simulink model "MINI_BANSHEE_bckup"  (Simulink 8.1)
settings: Solver=ode1  StartTime=0.0  StopTime=inf  FixedStep=Ts  MaxStep=1e-3  RelTol=1e-3
PostLoadFcn:
  | BANSHEE_init;
InitFcn:
  | BANSHEE_init;
undefined symbols (not defined in the file): cable_spec, F1, F2, F3, fdesignblkfcn, gcbh, Left, SM_UtilityService, Ts, type, utility_service_lib, V
libraries: rtio_generic_modbus x37, relay_modbus_lib x36, cables_lib x17, breaker_lib x17, rtlab x15, rtio_opalrt_common x15, artemis x11, simulink x10, transformer_lib x7, simulink_extras x6, PQFV_lib x5, rtio_opalrt_op5142ex1 x4
(part 2 of 3)

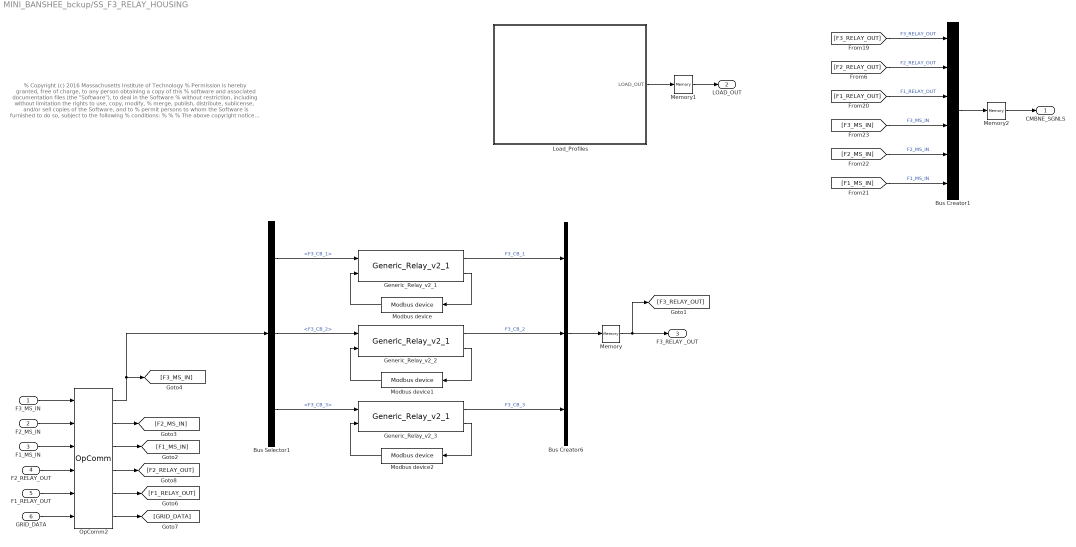
== system MINI_BANSHEE_bckup/SS_F3_RELAY_HOUSING ==
  note: % Copyright (c) 2016 Massachusetts Institute of Technology
      | % Permission is hereby granted, free of charge, to any person obtaining a copy of this
      | % software and associated documentation files (the "Software"), to deal in the Software
      | % without restriction, including without limitation the rights to use, copy, modify,
      | % merge, publish, distribute, sublicense, and/or sell copies of the Software, and to
      | % permit persons to whom the Software is furnished to do so, subject to the following
      | % conditions:
      | %
      | %
      | % The above copyright notice and this permission notice shall be included in
      | % all copies or substantial portions of the Software.
      | %
      | % THE SOFTWARE IS PROVIDED "AS IS", WITHOUT WARRANTY OF ANY KIND, EXPRESS OR IMPLIED,
      | % INCLUDING BUT NOT LIMITED TO THE WARRANTIES OF MERCHANTABILITY, FITNESS FOR A
      | % PARTICULAR PURPOSE AND NONINFRINGEMENT. IN NO EVENT SHALL THE AUTHORS OR COPYRIGHT
      | % HOLDERS BE LIABLE FOR ANY CLAIM, DAMAGES OR OTHER LIABILITY, WHETHER IN AN ACTION
      | % OF CONTRACT, TORT OR OTHERWISE, ARISING FROM, OUT OF OR IN CONNECTION WITH THE
      | % SOFTWARE OR THE USE OR OTHER DEALINGS IN THE SOFTWARE.
      | %
      | %
      | %%
  F3_MS_IN : Inport
  F2_MS_IN : Inport  Port=2
  F1_MS_IN : Inport  Port=3
  F2_RELAY_OUT : Inport  Port=4
  F1_RELAY_OUT : Inport  Port=5
  GRID_DATA : Inport  Port=6
  Bus Creator1 : BusCreator  Inputs=6
  Bus Creator6 : BusCreator  Inputs=3
  Bus Selector1 : BusSelector  OutputSignals=CB_DATA.F3_CB_1,CB_DATA.F3_CB_2,CB_DATA.F3_CB_3
  Generic_Relay_v2_1 : relay_modbus_lib/Generic_Relay_v2_1  Ts=Ts  relay_settings=[F3(1,:)]
  Generic_Relay_v2_2 : relay_modbus_lib/Generic_Relay_v2_1  Ts=Ts  relay_settings=[F3(2,:)]
  Generic_Relay_v2_3 : relay_modbus_lib/Generic_Relay_v2_1  Ts=Ts  relay_settings=[F3(3,:)]
  Load_Profiles : Subsystem
  Memory : Memory
  Memory1 : Memory
  Memory2 : Memory
  Modbus device : rtio_generic_modbus/Modbus device  conf_name=F3_relay_cfg1.opal  conf_name_mask=F3_relay_cfg1.xls  sample_time=Ts
  Modbus device1 : rtio_generic_modbus/Modbus device  conf_name=F3_relay_cfg2.opal  conf_name_mask=F3_relay_cfg2.xls  sample_time=Ts
  Modbus device2 : rtio_generic_modbus/Modbus device  conf_name=F3_relay_cfg3.opal  conf_name_mask=F3_relay_cfg3.xls  sample_time=Ts
  OpComm2 : rtlab/OpComm  nbport=6  groupe_acq=1  subsys_rate=0  st=0  Synchronization=on  Interpolation=on  Threshold=1.0  Missed_Data=off  Sim_Time=off  Samples=off  dynSigOut=off  from_console=0  warning_done=off  writeOpCommFile=off  Offset=off
  CMBNE_SGNLS : Outport
  LOAD_OUT : Outport  Port=2
  F3_RELAY _OUT : Outport  Port=3
  wires:
  Load_Profiles/1(LOAD_OUT) -> Memory1/1
  OpComm2/1 -> Bus Selector1/1, [F3_MS_IN]
  Generic_Relay_v2_1/2 -> Modbus device/1
  Modbus device/1 -> Generic_Relay_v2_1/2
  Generic_Relay_v2_2/2 -> Modbus device1/1
  Modbus device1/1 -> Generic_Relay_v2_2/2
  Modbus device2/1 -> Generic_Relay_v2_3/2
  Generic_Relay_v2_3/2 -> Modbus device2/1
  F3_MS_IN/1 -> OpComm2/1
  Bus Selector1/1 -> Generic_Relay_v2_1/1  "<F3_CB_1>"
  Bus Selector1/2 -> Generic_Relay_v2_2/1  "<F3_CB_2>"
  Bus Selector1/3 -> Generic_Relay_v2_3/1  "<F3_CB_3>"
  Generic_Relay_v2_1/1 -> Bus Creator6/1  "F3_CB_1"
  Generic_Relay_v2_2/1 -> Bus Creator6/2  "F3_CB_2"
  Generic_Relay_v2_3/1 -> Bus Creator6/3  "F3_CB_3"
  Bus Creator6/1 -> Memory/1
  Memory/1 -> [F3_RELAY_OUT], F3_RELAY _OUT/1
  Memory1/1 -> LOAD_OUT/1
  F2_RELAY_OUT/1 -> OpComm2/4
  F1_RELAY_OUT/1 -> OpComm2/5
  OpComm2/4 -> [F2_RELAY_OUT]
  OpComm2/5 -> [F1_RELAY_OUT]
  OpComm2/2 -> [F2_MS_IN]
  OpComm2/3 -> [F1_MS_IN]
  F2_MS_IN/1 -> OpComm2/2
  F1_MS_IN/1 -> OpComm2/3
  OpComm2/6 -> [GRID_DATA]
  GRID_DATA/1 -> OpComm2/6
  Memory2/1 -> CMBNE_SGNLS/1
  Bus Creator1/1 -> Memory2/1
  [F1_MS_IN] -> Bus Creator1/6  "F1_MS_IN"
  [F2_RELAY_OUT] -> Bus Creator1/2  "F2_RELAY_OUT"
  [F1_RELAY_OUT] -> Bus Creator1/3  "F1_RELAY_OUT"
  [F3_RELAY_OUT] -> Bus Creator1/1  "F3_RELAY_OUT"
  [F3_MS_IN] -> Bus Creator1/4  "F3_MS_IN"
  [F2_MS_IN] -> Bus Creator1/5  "F2_MS_IN"

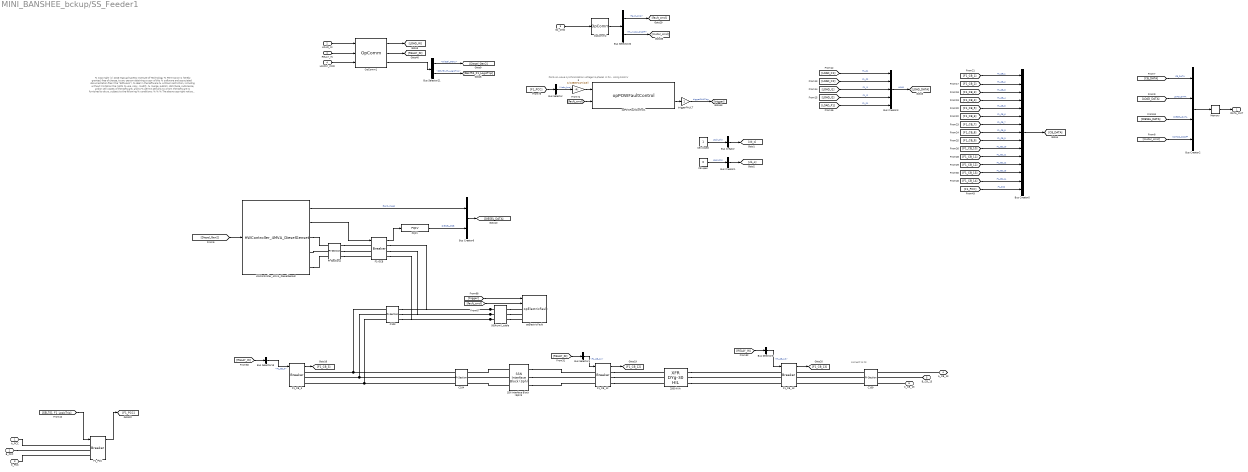
== system MINI_BANSHEE_bckup/SS_Feeder1 ==
  note: connect to F3
  note: % Copyright (c) 2016 Massachusetts Institute of Technology
      | % Permission is hereby granted, free of charge, to any person obtaining a copy of this
      | % software and associated documentation files (the "Software"), to deal in the Software
      | % without restriction, including without limitation the rights to use, copy, modify,
      | % merge, publish, distribute, sublicense, and/or sell copies of the Software, and to
      | % permit persons to whom the Software is furnished to do so, subject to the following
      | % conditions:
      | %
      | %
      | % The above copyright notice and this permission notice shall be included in
      | % all copies or substantial portions of the Software.
      | %
      | % THE SOFTWARE IS PROVIDED "AS IS", WITHOUT WARRANTY OF ANY KIND, EXPRESS OR IMPLIED,
      | % INCLUDING BUT NOT LIMITED TO THE WARRANTIES OF MERCHANTABILITY, FITNESS FOR A
      | % PARTICULAR PURPOSE AND NONINFRINGEMENT. IN NO EVENT SHALL THE AUTHORS OR COPYRIGHT
      | % HOLDERS BE LIABLE FOR ANY CLAIM, DAMAGES OR OTHER LIABILITY, WHETHER IN AN ACTION
      | % OF CONTRACT, TORT OR OTHERWISE, ARISING FROM, OUT OF OR IN CONNECTION WITH THE
      | % SOFTWARE OR THE USE OR OTHER DEALINGS IN THE SOFTWARE.
      | %
      | %
      | %%
  note: Point-on-wave synchronisation voltage (3-phase) in PU - Using 13.8 kV
  RELAY_IN : Inport
  LOAD_IN : Inport  Port=2
  SC_CMD : Inport  Port=3
  HWCtrl_CMD : Inport  Port=4
  2500 kVA : transformer_lib/XFR DYg-30 HIL  Rating=2500  Vp=13800  Vs=480  Z=5.75  XR=6.6
  500kcmil_cable : cables_lib/500kcmil_cable  length=1  par_sets=1
  Bus Creator : BusCreator  Inputs=1
  Bus Creator1 : BusCreator  Inputs=1
  Bus Creator2 : BusCreator
  Bus Creator3 : BusCreator  Inputs=5
  Bus Creator5 : BusCreator  Inputs=15
  Bus Creator6 : BusCreator  Inputs=2
  Bus Selector : BusSelector  OutputSignals=Vabc_bus
  Bus Selector1 : BusSelector  OutputSignals=F1_CB_12
  Bus Selector13 : BusSelector  OutputSignals=F1_CB_3
  Bus Selector20 : BusSelector  OutputSignals=fault_cmd,motor_ONOFF.F1_motor_ONOFF
  Bus Selector21 : BusSelector  OutputSignals=Diesel_Gen2,SEL751-F1_LogicTrip
  Bus Selector8 : BusSelector  OutputSignals=F1_CB_13
  C103 : cables_lib/PI-Section  cable_spec=[cable_spec(11, :)]  line_length=1000  parallel_sets=1
  C104 : cables_lib/PI-Section  cable_spec=[cable_spec(13, :)]  line_length=3000  parallel_sets=1
  C109 : cables_lib/PI-Section  cable_spec=[cable_spec(6, :)]  line_length=2000  parallel_sets=2
  CB closed : Constant
  CB open : Constant  Value=0
  F1-GCB : breaker_lib/Breaker  Ts=Ts  mech_delay=cb_mech_delay
  F1_CB_12 : breaker_lib/Breaker  Ts=Ts  mech_delay=cb_mech_delay
  F1_CB_13 : breaker_lib/Breaker  Ts=Ts  mech_delay=cb_mech_delay
  F1_CB_3 : breaker_lib/Breaker  Ts=Ts  mech_delay=cb_mech_delay
  F1_PCC : breaker_lib/Breaker  Ts=Ts  mech_delay=cb_mech_delay
  HWController_4MVA_DieselGenset : HWController_Diesel_GenSet_4MVA_lib/HWController_4MVA_DieselGenset
  Memory : Memory
  OpComm1 : rtlab/OpComm  nbport=3  groupe_acq=1  subsys_rate=0  st=0  Synchronization=on  Interpolation=on  Threshold=1.0  Missed_Data=off  Sim_Time=off  Samples=off  dynSigOut=off  from_console=0  warning_done=off  writeOpCommFile=off  Offset=off
  OpComm2 : rtlab/OpComm  nbport=1  groupe_acq=1  subsys_rate=0  st=0  Synchronization=on  Interpolation=on  Threshold=1.0  Missed_Data=off  Sim_Time=off  Samples=off  dynSigOut=off  from_console=1  warning_done=off  writeOpCommFile=off  Offset=off
  PI-Section4 : cables_lib/PI-Section  cable_spec=[cable_spec(11, :)]  line_length=2000  parallel_sets=1
  PQFV : PQFV_lib/PQFV  VRMSLL=13800
  SSN Interface Block (3ph)3 : ssn_lib/SSN Interface Block (3ph)  nb_phase=3  nb_port=2  p1_type=V-type(Left)  p2_type=V-type (Right)  p3_type=V-type(Left)  p4_type=V-type(Left)  p5_type=V-type(Left)  p6_type=V-type(Left)  p7_type=V-type(Left)  p8_type=V-type(Left)  p9_type=V-type(Left)  p10_type=V-type(Left)  p11_type=V-type(Left)  p12_type=V-type(Left)  p13_type=V-type(Left)  p14_type=V-type(Left)  p15_type=V-type(Left)  p16_type=V-type(Left)  I_port_shunt_resistance=1e9
  a : Gain  Gain=1/(13800*sqrt(2/3))
  opElectricFault : artemis/Tools /POW faults/opElectricFault  FaultLocation=location 2  FaultResistance=0.0001  GroundResistance=0.0001  InitialStates=[0 0 0]  SnubberResistance=1e6  SnubberCapacitance=inf
  opPOWFaultControl1 : artemis/Tools /POW faults/opPOWFaultControl  Ts=Ts  usePLL=off  Fgrid=60  PLL_k=[180 3200 1]  vol_sel=1: rising zero-corssing  SyncPhase_menu=A  T_acq=0.8
  triggerFAULT : Gain
  A_PCC : PMIOPort  Port=1  Side=Left
  B_PCC : PMIOPort  Port=2  Side=Left
  C_PCC : PMIOPort  Port=3  Side=Left
  A_CB_13 : PMIOPort  Port=4  Side=Right
  B_CB_13 : PMIOPort  Port=5  Side=Right
  C_CB_13 : PMIOPort  Port=6  Side=Right
  DATA_OUT : Outport
  wires:
  F1_PCC/1 -> [F1_PCC]
  Bus Creator/1 -> [cb_c]
  CB closed/1 -> Bus Creator/1  "Logic_trip"
  Bus Creator1/1 -> [cb_o]
  CB open/1 -> Bus Creator1/1  "Logic_trip"
  LOAD_IN/1 -> OpComm1/1
  OpComm1/1 -> [LOAD_IN]
  [LOAD_C1] -> Bus Creator3/1  "F1_C1"
  [LOAD_I2] -> Bus Creator3/4  "F1_I2"
  [LOAD_P1] -> Bus Creator3/5  "F1_P1"
  [LOAD_C2] -> Bus Creator3/2  "F1_C2"
  [LOAD_I1] -> Bus Creator3/3  "F1_I1"
  F1_CB_3/1 -> [F1_CB_3]
  F1_CB_12/1 -> [F1_CB_12]
  F1_CB_13/1 -> [F1_CB_13]
  [F1_CB_1] -> Bus Creator5/1  "F1_CB_1"
  [F1_CB_13] -> Bus Creator5/13  "F1_CB_13"
  [F1_CB_12] -> Bus Creator5/12  "F1_CB_12"
  [F1_CB_11] -> Bus Creator5/11  "F1_CB_11"
  [F1_CB_10] -> Bus Creator5/10  "F1_CB_10"
  [F1_CB_9] -> Bus Creator5/9  "F1_CB_9"
  [F1_CB_8] -> Bus Creator5/8  "F1_CB_8"
  [F1_CB_7] -> Bus Creator5/7  "F1_CB_7"
  [F1_CB_6] -> Bus Creator5/6  "F1_CB_6"
  [F1_CB_5] -> Bus Creator5/5  "F1_CB_5"
  [F1_CB_4] -> Bus Creator5/4  "F1_CB_4"
  [F1_CB_3] -> Bus Creator5/3  "F1_CB_3"
  [F1_CB_2] -> Bus Creator5/2  "F1_CB_2"
  RELAY_IN/1 -> OpComm1/2
  OpComm1/2 -> [RELAY_IN]
  Bus Selector13/1 -> F1_CB_3/1  "<F1_CB_3>"
  [RELAY_IN] -> Bus Selector13/1
  [RELAY_IN] -> Bus Selector1/1
  [RELAY_IN] -> Bus Selector8/1
  Bus Selector1/1 -> F1_CB_12/1  "<F1_CB_12>"
  Bus Selector8/1 -> F1_CB_13/1  "<F1_CB_13>"
  [F1_PCC] -> Bus Creator5/15  "F1_PCC"
  [F1_CB_14] -> Bus Creator5/14  "F1_CB_14"
  [fault_cmd] -> opPOWFaultControl1/2
  opPOWFaultControl1/2 -> triggerFAULT/1
  triggerFAULT/1 -> [trigger]  "triggerFAULTsig"
  [F1_PCC] -> Bus Selector/1
  Bus Selector/1 -> a/1  "<Vabc_bus>"
  a/1 -> opPOWFaultControl1/1
  SC_CMD/1 -> OpComm2/1
  [fault_cmd] -> opElectricFault/2
  [trigger] -> opElectricFault/1
  OpComm2/1 -> Bus Selector20/1
  Bus Selector20/1 -> [fault_cmd]  "<fault_cmd>"
  Bus Creator3/1 -> [LOAD_DATA]  "LOAD"
  Bus Creator5/1 -> [CB_DATA]
  [Diesel_Gen2] -> HWController_4MVA_DieselGenset/1
  HWController_4MVA_DieselGenset/2 -> F1-GCB/1
  OpComm1/3 -> Bus Selector21/1
  Bus Selector21/1 -> [Diesel_Gen2]  "<Diesel_Gen2>"
  HWCtrl_CMD/1 -> OpComm1/3
  F1-GCB/1 -> PQFV/1
  Bus Creator6/1 -> [DIESEL_DATA]
  PQFV/1 -> Bus Creator6/2  "DIESEL_GCB"
  HWController_4MVA_DieselGenset/1 -> Bus Creator6/1  "Gen2_meas"
  Memory/1 -> DATA_OUT/1
  Bus Creator2/1 -> Memory/1
  [CB_DATA] -> Bus Creator2/1  "CB_DATA"
  [LOAD_DATA] -> Bus Creator2/2  "LOAD_DATA"
  [DIESEL_DATA] -> Bus Creator2/3  "DIESEL_DATA"
  Bus Selector20/2 -> [motor_cmd]  "<F1_motor_ONOFF>"
  [motor_cmd] -> Bus Creator2/4  "MOTOR_ONOFF"
  Bus Selector21/2 -> [SEL751_F1_LogicTrip]  "<SEL751-F1_LogicTrip>"
  [SEL751_F1_LogicTrip] -> F1_PCC/1
  connections:
  2500 kVA/RConn2 -- F1_CB_13/LConn2
  F1_CB_12/RConn1 -- 2500 kVA/LConn1
  A_PCC/RConn1 -- F1_PCC/LConn1
  B_PCC/RConn1 -- F1_PCC/LConn2
  C104/LConn2 -- C103/LConn2 -- F1_CB_3/RConn2
  F1_CB_12/RConn2 -- 2500 kVA/LConn2
  F1_CB_12/RConn3 -- 2500 kVA/LConn3
  C104/LConn1 -- C103/LConn1 -- F1_CB_3/RConn1
  C104/LConn3 -- C103/LConn3 -- F1_CB_3/RConn3
  2500 kVA/RConn1 -- F1_CB_13/LConn1
  C_PCC/RConn1 -- F1_PCC/LConn3
  2500 kVA/RConn3 -- F1_CB_13/LConn3
  C109/LConn1 -- F1_CB_13/RConn1
  C109/LConn3 -- F1_CB_13/RConn3
  C109/LConn2 -- F1_CB_13/RConn2
  C_CB_13/RConn1 -- C109/RConn3
  B_CB_13/RConn1 -- C109/RConn2
  A_CB_13/RConn1 -- C109/RConn1
  SSN Interface Block (3ph)3/LConn2 -- C104/RConn2
  SSN Interface Block (3ph)3/LConn3 -- C104/RConn3
  SSN Interface Block (3ph)3/LConn1 -- C104/RConn1
  SSN Interface Block (3ph)3/RConn2 -- F1_CB_12/LConn2
  SSN Interface Block (3ph)3/RConn1 -- F1_CB_12/LConn1
  SSN Interface Block (3ph)3/RConn3 -- F1_CB_12/LConn3
  500kcmil_cable/RConn3 -- opElectricFault/LConn3
  500kcmil_cable/RConn1 -- opElectricFault/LConn1
  500kcmil_cable/RConn2 -- opElectricFault/LConn2
  500kcmil_cable/LConn3 -- C103/RConn3 -- F1-GCB/RConn3
  500kcmil_cable/LConn2 -- C103/RConn2 -- F1-GCB/RConn2
  500kcmil_cable/LConn1 -- C103/RConn1 -- F1-GCB/RConn1
  PI-Section4/RConn3 -- F1-GCB/LConn3
  PI-Section4/RConn1 -- F1-GCB/LConn1
  PI-Section4/RConn2 -- F1-GCB/LConn2
  HWController_4MVA_DieselGenset/RConn1 -- PI-Section4/LConn1
  HWController_4MVA_DieselGenset/RConn2 -- PI-Section4/LConn2
  HWController_4MVA_DieselGenset/RConn3 -- PI-Section4/LConn3

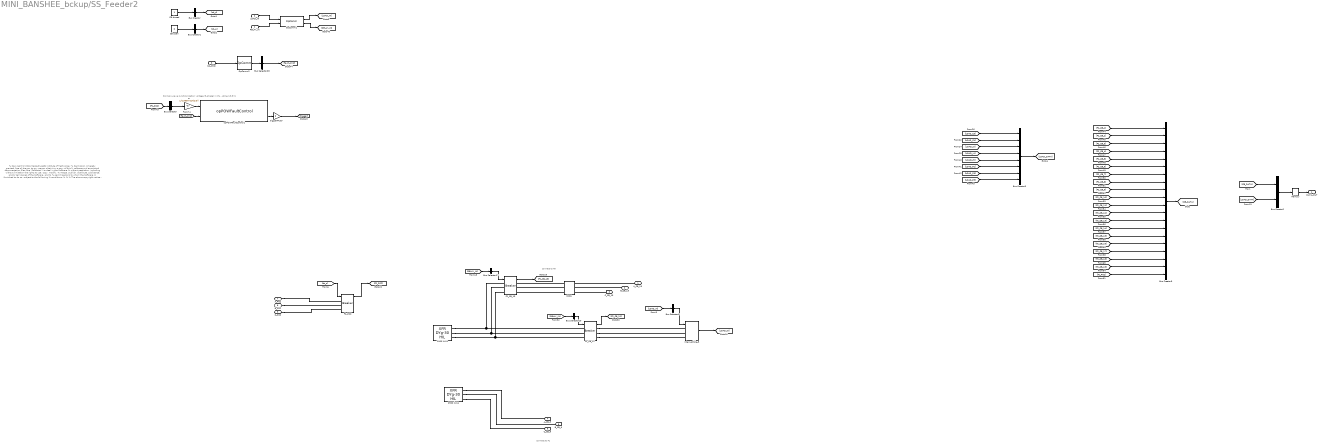
== system MINI_BANSHEE_bckup/SS_Feeder2 ==
  note: connect to F3
  note: connect to F1
  note: % Copyright (c) 2016 Massachusetts Institute of Technology
      | % Permission is hereby granted, free of charge, to any person obtaining a copy of this
      | % software and associated documentation files (the "Software"), to deal in the Software
      | % without restriction, including without limitation the rights to use, copy, modify,
      | % merge, publish, distribute, sublicense, and/or sell copies of the Software, and to
      | % permit persons to whom the Software is furnished to do so, subject to the following
      | % conditions:
      | %
      | %
      | % The above copyright notice and this permission notice shall be included in
      | % all copies or substantial portions of the Software.
      | %
      | % THE SOFTWARE IS PROVIDED "AS IS", WITHOUT WARRANTY OF ANY KIND, EXPRESS OR IMPLIED,
      | % INCLUDING BUT NOT LIMITED TO THE WARRANTIES OF MERCHANTABILITY, FITNESS FOR A
      | % PARTICULAR PURPOSE AND NONINFRINGEMENT. IN NO EVENT SHALL THE AUTHORS OR COPYRIGHT
      | % HOLDERS BE LIABLE FOR ANY CLAIM, DAMAGES OR OTHER LIABILITY, WHETHER IN AN ACTION
      | % OF CONTRACT, TORT OR OTHERWISE, ARISING FROM, OUT OF OR IN CONNECTION WITH THE
      | % SOFTWARE OR THE USE OR OTHER DEALINGS IN THE SOFTWARE.
      | %
      | %
      | %%
  note: Point-on-wave synchronisation voltage (3-phase) in PU - Using 13.8 kV
  RELAY_IN : Inport
  LOAD_IN : Inport  Port=2
  SC_CMD : Inport  Port=3
  1000 kVA1 : transformer_lib/XFR DYg-30 HIL  Rating=1000  Vp=13800  Vs=480  Z=5.56  XR=4.49
  2500 kVA1 : transformer_lib/XFR DYg-30 HIL  Rating=2500  Vp=13800  Vs=480  Z=5.56  XR=5.52
  Bus Creator : BusCreator  Inputs=1
  Bus Creator1 : BusCreator  Inputs=1
  Bus Creator2 : BusCreator  Inputs=2
  Bus Creator3 : BusCreator  Inputs=8
  Bus Creator5 : BusCreator  Inputs=20
  Bus Selector : BusSelector  OutputSignals=Vabc_bus
  Bus Selector17 : BusSelector  OutputSignals=F2_CB_13
  Bus Selector20 : BusSelector  OutputSignals=F2_CB_12
  Bus Selector28 : BusSelector  OutputSignals=fault_cmd
  Bus Selector5 : BusSelector  OutputSignals=I5
  C206 : cables_lib/PI-Section  cable_spec=[cable_spec(6, :)]  line_length=1500  parallel_sets=2
  CB closed : Constant
  CB open : Constant  Value=0
  F2_CB_12 : breaker_lib/Breaker  Ts=Ts  mech_delay=cb_mech_delay
  F2_CB_13 : breaker_lib/Breaker  Ts=Ts  mech_delay=cb_mech_delay
  F2_PCC : breaker_lib/Breaker  Ts=Ts  mech_delay=cb_mech_delay
  Interruptible_5 : Load_lib/Dynamic_Load  V=460  Ts=Ts
  Memory : Memory
  OpComm1 : rtlab/OpComm  nbport=2  groupe_acq=1  subsys_rate=0  st=0  Synchronization=on  Interpolation=on  Threshold=1.0  Missed_Data=off  Sim_Time=off  Samples=off  dynSigOut=off  from_console=0  warning_done=off  writeOpCommFile=off  Offset=off
  OpComm2 : rtlab/OpComm  nbport=1  groupe_acq=1  subsys_rate=0  st=0  Synchronization=on  Interpolation=on  Threshold=1.0  Missed_Data=off  Sim_Time=off  Samples=off  dynSigOut=off  from_console=1  warning_done=off  writeOpCommFile=off  Offset=off
  a : Gain  Gain=1/(13800*sqrt(2/3))
  opPOWFaultControl1 : artemis/Tools /POW faults/opPOWFaultControl  Ts=Ts  usePLL=off  Fgrid=60  PLL_k=[180 3200 1]  vol_sel=1: rising zero-corssing  SyncPhase_menu=A  T_acq=0.8
  triggerFAULT : Gain
  A_CB_13 : PMIOPort  Port=1  Side=Right
  B_CB_13 : PMIOPort  Port=2  Side=Right
  C_CB_13 : PMIOPort  Port=3  Side=Right
  A_CB_9 : PMIOPort  Port=4  Side=Right
  B_CB_9 : PMIOPort  Port=5  Side=Right
  C_CB_9 : PMIOPort  Port=6  Side=Right
  A_PCC : PMIOPort  Port=7  Side=Left
  B_PCC : PMIOPort  Port=8  Side=Left
  C_PCC : PMIOPort  Port=9  Side=Left
  DATA_OUT : Outport
  wires:
  [cb_c] -> F2_PCC/1
  Bus Creator/1 -> [cb_c]
  CB closed/1 -> Bus Creator/1  "Logic_trip"
  Bus Creator1/1 -> [cb_o]
  CB open/1 -> Bus Creator1/1  "Logic_trip"
  LOAD_IN/1 -> OpComm1/1
  OpComm1/1 -> [LOAD_IN]
  [LOAD_IN] -> Bus Selector5/1
  Bus Selector5/1 -> Interruptible_5/1  "<I5>"
  Interruptible_5/1 -> [LOAD_I5]
  [LOAD_C3] -> Bus Creator3/1  "F2_C3"
  Bus Creator3/1 -> [LOAD_DATA]  "LOAD"
  [LOAD_I4] -> Bus Creator3/4  "F2_I4"
  [LOAD_P2] -> Bus Creator3/6  "F2_P2"
  [LOAD_I5] -> Bus Creator3/5  "F2_I5"
  [LOAD_C4] -> Bus Creator3/2  "F2_C4"
  [LOAD_I3] -> Bus Creator3/3  "F2_I3"
  [LOAD_P3] -> Bus Creator3/7  "F2_P3"
  [LOAD_P5] -> Bus Creator3/8  "F2_P5"
  F2_CB_13/1 -> [F2_CB_13]
  [F2_CB_1] -> Bus Creator5/1  "F2_CB_1"
  [F2_CB_2] -> Bus Creator5/2  "F2_CB_2"
  [F2_CB_3] -> Bus Creator5/3  "F2_CB_3"
  [F2_CB_6] -> Bus Creator5/6  "F2_CB_6"
  [F2_CB_4] -> Bus Creator5/4  "F2_CB_4"
  [F2_CB_9] -> Bus Creator5/9  "F2_CB_9"
  [F2_CB_7] -> Bus Creator5/7  "F2_CB_7"
  [F2_CB_11] -> Bus Creator5/11  "F2_CB_11"
  [F2_CB_14] -> Bus Creator5/14  "F2_CB_14"
  [F2_CB_5] -> Bus Creator5/5  "F2_CB_5"
  [F2_CB_8] -> Bus Creator5/8  "F2_CB_8"
  [F2_CB_12] -> Bus Creator5/12  "F2_CB_12"
  [F2_CB_10] -> Bus Creator5/10  "F2_CB_10"
  [F2_CB_13] -> Bus Creator5/13  "F2_CB_13"
  [F2_CB_15] -> Bus Creator5/15  "F2_CB_15"
  [F2_CB_16] -> Bus Creator5/16  "F2_CB_16"
  RELAY_IN/1 -> OpComm1/2
  OpComm1/2 -> [RELAY_IN]
  [RELAY_IN] -> Bus Selector17/1
  [RELAY_IN] -> Bus Selector20/1
  Bus Selector17/1 -> F2_CB_13/1  "<F2_CB_13>"
  Bus Selector20/1 -> F2_CB_12/1  "<F2_CB_12>"
  [F2_CB_17] -> Bus Creator5/17  "F2_CB_17"
  F2_CB_12/1 -> [F2_CB_12]
  F2_PCC/1 -> [F2_PCC]
  [F2_PCC] -> Bus Creator5/20  "F2_PCC"
  [F2_CB_18] -> Bus Creator5/18  "F2_CB_18"
  [F2_CB_19] -> Bus Creator5/19  "F2_CB_19"
  [fault_cmd] -> opPOWFaultControl1/2
  opPOWFaultControl1/2 -> triggerFAULT/1
  triggerFAULT/1 -> [trigger]  "triggerFAULTsig"
  [F2_PCC] -> Bus Selector/1
  Bus Selector/1 -> a/1  "<Vabc_bus>"
  a/1 -> opPOWFaultControl1/1
  SC_CMD/1 -> OpComm2/1
  Memory/1 -> DATA_OUT/1
  OpComm2/1 -> Bus Selector28/1
  Bus Selector28/1 -> [fault_cmd]  "<fault_cmd>"
  Bus Creator2/1 -> Memory/1
  Bus Creator5/1 -> [CB_DATA]
  [CB_DATA] -> Bus Creator2/1  "CB_DATA"
  [LOAD_DATA] -> Bus Creator2/2  "LOAD_DATA"
  connections:
  F2_CB_13/LConn1 -- F2_CB_12/LConn1 -- 1000 kVA1/RConn1
  F2_CB_13/LConn2 -- 1000 kVA1/RConn2 -- F2_CB_12/LConn2
  F2_CB_13/LConn3 -- F2_CB_12/LConn3 -- 1000 kVA1/RConn3
  F2_CB_12/RConn3 -- Interruptible_5/LConn3
  F2_CB_12/RConn2 -- Interruptible_5/LConn2
  F2_CB_12/RConn1 -- Interruptible_5/LConn1
  C_PCC/RConn1 -- F2_PCC/LConn3
  B_PCC/RConn1 -- F2_PCC/LConn2
  A_PCC/RConn1 -- F2_PCC/LConn1
  2500 kVA1/RConn2 -- B_CB_9/RConn1
  2500 kVA1/RConn1 -- A_CB_9/RConn1
  2500 kVA1/RConn3 -- C_CB_9/RConn1
  C206/LConn3 -- F2_CB_13/RConn3
  C206/LConn2 -- F2_CB_13/RConn2
  C206/LConn1 -- F2_CB_13/RConn1
  C_CB_13/RConn1 -- C206/RConn3
  B_CB_13/RConn1 -- C206/RConn2
  A_CB_13/RConn1 -- C206/RConn1

== system MINI_BANSHEE_bckup/SC_ctrl/Overall ==
  F1 : Inport
  F2 : Inport  Port=2
  F3 : Inport  Port=3
  Iabc : Scope  NumInputPorts=3
      settings: ShowLegends=on  TimeRange=10  YMin=0~0~2  YMax=47.5~650~21  Decimation=10
  Vpu : Scope  NumInputPorts=3
      settings: ShowLegends=on  TimeRange=10  YMin=0.9975~1.0125~0.955  YMax=1.055~1.0675~1.06  SaveName=ScopeData3  Decimation=10
  currents : Subsystem
  voltages : Subsystem
  wires:
  voltages/1(oF1) -> Vpu/1
  voltages/2(oF2) -> Vpu/2
  voltages/3(oF3) -> Vpu/3
  currents/1(oF1) -> Iabc/1
  currents/2(oF2) -> Iabc/2
  currents/3(oF3) -> Iabc/3
  F3/1 -> voltages/3(F3), currents/3(F3)
  F2/1 -> currents/2(F2), voltages/2(F2)
  F1/1 -> voltages/1(F1), currents/1(F1)

== system MINI_BANSHEE_bckup/SC_ctrl/Status ==
  F1 : Inport
  F2 : Inport  Port=2
  F3 : Inport  Port=3
  Bus Selector : BusSelector  OutputSignals=F1_CB_1.m.status,F1_CB_2.m.status,F1_CB_3.m.status,F1_CB_4.m.status,F1_CB_5.m.status,F1_CB_6.m.status,F1_CB_7.m.status,F1_CB_8.m.status,F1_CB_9.m.status,F1_CB_10.m.status,F1_CB_11.m.status,F1_CB_12.m.status,F1_CB_13.m.status,F1_CB_14.m.status
  Bus Selector1 : BusSelector  OutputSignals=F2_CB_1.m.status,F2_CB_2.m.status,F2_CB_3.m.status,F2_CB_4.m.status,F2_CB_5.m.status,F2_CB_6.m.status,F2_CB_7.m.status,F2_CB_8.m.status,F2_CB_9.m.status,F2_CB_10.m.status,F2_CB_11.m.status,F2_CB_12.m.status,F2_CB_13.m.status,F2_CB_14.m.status,F2_CB_15.m.status,F2_CB_16.m.status,F2_CB_17.m.status,F2_CB_18.m.status,F2_CB_19.m.status
  Bus Selector2 : BusSelector  OutputSignals=F3_CB_1.m.status,F3_CB_2.m.status,F3_CB_3.m.status,F3_CB_4.m.status,F3_CB_5.m.status,F3_CB_6.m.status,F3_CB_7.m.status,F3_CB_8.m.status,F3_CB_9.m.status
  Mux : Mux  Inputs=14
  Mux1 : Mux  Inputs=19
  Mux2 : Mux  Inputs=9
  Status : Scope  NumInputPorts=3
      settings: ShowLegends=on  TimeRange=0.4  YMin=2~2~3  YMax=3~3~3  SaveName=ScopeData3  Decimation=20
  wires:
  Mux/1 -> Status/1  "F1"
  F1/1 -> Bus Selector/1
  Mux1/1 -> Status/2  "F2"
  F2/1 -> Bus Selector1/1
  Mux2/1 -> Status/3  "F3"
  F3/1 -> Bus Selector2/1
  Bus Selector1/3 -> Mux1/3  "<status>"
  Bus Selector1/13 -> Mux1/13  "<status>"
  Bus Selector1/8 -> Mux1/8  "<status>"
  Bus Selector1/4 -> Mux1/4  "<status>"
  Bus Selector1/6 -> Mux1/6  "<status>"
  Bus Selector1/2 -> Mux1/2  "<status>"
  Bus Selector1/7 -> Mux1/7  "<status>"
  Bus Selector1/10 -> Mux1/10  "<status>"
  Bus Selector1/12 -> Mux1/12  "<status>"
  Bus Selector1/1 -> Mux1/1  "<status>"
  Bus Selector1/5 -> Mux1/5  "<status>"
  Bus Selector1/14 -> Mux1/14  "<status>"
  Bus Selector1/9 -> Mux1/9  "<status>"
  Bus Selector1/11 -> Mux1/11  "<status>"
  Bus Selector1/17 -> Mux1/17  "<status>"
  Bus Selector1/16 -> Mux1/16  "<status>"
  Bus Selector1/15 -> Mux1/15  "<status>"
  Bus Selector1/18 -> Mux1/18  "<status>"
  Bus Selector1/19 -> Mux1/19  "<status>"
  Bus Selector/4 -> Mux/4  "<status>"
  Bus Selector/10 -> Mux/10  "<status>"
  Bus Selector/8 -> Mux/8  "<status>"
  Bus Selector/1 -> Mux/1  "<status>"
  Bus Selector/7 -> Mux/7  "<status>"
  Bus Selector/12 -> Mux/12  "<status>"
  Bus Selector/5 -> Mux/5  "<status>"
  Bus Selector/9 -> Mux/9  "<status>"
  Bus Selector/2 -> Mux/2  "<status>"
  Bus Selector/3 -> Mux/3  "<status>"
  Bus Selector/6 -> Mux/6  "<status>"
  Bus Selector/11 -> Mux/11  "<status>"
  Bus Selector/13 -> Mux/13  "<status>"
  Bus Selector/14 -> Mux/14  "<status>"
  Bus Selector2/6 -> Mux2/6  "<status>"
  Bus Selector2/5 -> Mux2/5  "<status>"
  Bus Selector2/7 -> Mux2/7  "<status>"
  Bus Selector2/4 -> Mux2/4  "<status>"
  Bus Selector2/8 -> Mux2/8  "<status>"
  Bus Selector2/3 -> Mux2/3  "<status>"
  Bus Selector2/9 -> Mux2/9  "<status>"
  Bus Selector2/2 -> Mux2/2  "<status>"
  Bus Selector2/1 -> Mux2/1  "<status>"

== system MINI_BANSHEE_bckup/SC_ctrl/Woodward ==
  16Din/16Dout GR3 : Subsystem
  Bus Creator2 : BusCreator  Inputs=1
  IOctrl : Outport
  wires:
  16Din/16Dout GR3/1(Dout) -> Bus Creator2/1  "16 DOUT GR3"
  Bus Creator2/1 -> IOctrl/1  "IO ctrl"

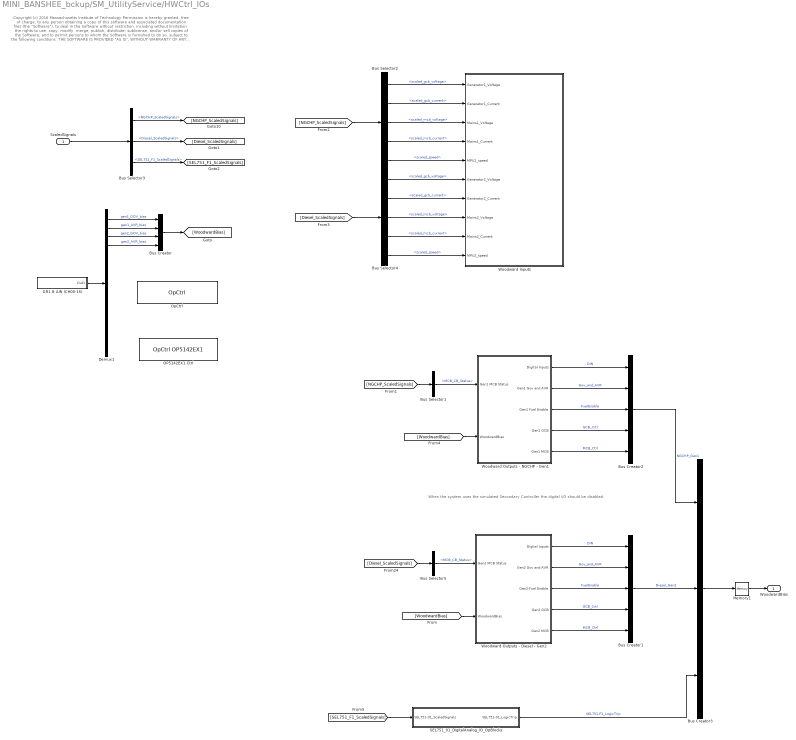
== system MINI_BANSHEE_bckup/SM_UtilityService/HWCtrl_IOs ==
  note: When the system uses the simulated
      | Secondary Controller the digital I/O
      | should be disabled.
  note: Copyright (c) 2016 Massachusetts Institute of Technology
      | Permission is hereby granted, free of charge, to any person obtaining a copy of this software and associated documentation files (the "Software"), to deal
      | in the Software without restriction, including without limitation the rights to use, copy, modify, merge, publish, distribute, sublicense, and/or sell copies of the
      | Software, and to permit persons to whom the Software is furnished to do so, subject to the following conditions:
      |
      | THE SOFTWARE IS PROVIDED "AS IS", WITHOUT WARRANTY OF ANY KIND, EXPRESS OR IMPLIED, INCLUDING BUT NOT LIMITED TO THE
      | WARRANTIES OF MERCHANTABILITY, FITNESS FOR A PARTICULAR PURPOSE AND NONINFRINGEMENT. IN NO EVENT SHALL THE AUTHORS
      | OR COPYRIGHT HOLDERS BE LIABLE FOR ANY CLAIM, DAMAGES OR OTHER LIABILITY, WHETHER IN AN ACTION OF CONTRACT, TORT OR
      | OTHERWISE, ARISING FROM, OUT OF OR IN CONNECTION WITH THE SOFTWARE OR THE USE OR OTHER DEALINGS IN THE SOFTWARE
  ScaledSignals : Inport
  Bus Creator : BusCreator
  Bus Creator1 : BusCreator  Inputs=5
  Bus Creator2 : BusCreator  Inputs=5
  Bus Creator3 : BusCreator  Inputs=3
  Bus Selector1 : BusSelector  OutputSignals=MCB_CB_Status
  Bus Selector2 : BusSelector  OutputSignals=scaled_gcb_voltage,scaled_gcb_current,scaled_mcb_voltage,scaled_mcb_current,scaled_speed
  Bus Selector3 : BusSelector  OutputSignals=NGCHP_ScaledSignals,Diesel_ScaledSignals,SEL751_F1_ScaledSignals
  Bus Selector4 : BusSelector  OutputSignals=scaled_gcb_voltage,scaled_gcb_current,scaled_mcb_voltage,scaled_mcb_current,scaled_speed
  Bus Selector5 : BusSelector  OutputSignals=MCB_CB_Status
  Demux1 : Demux  Outputs=16
  GR1 B AIN (CH00-15) : Subsystem
  Memory1 : Memory
  OP5142EX1 Ctrl : rtio_opalrt_op5142ex1/OpCtrl OP5142EX1  CtrlName='OP5142EX1 Ctrl'  boardid=1  BitstreamFilename=OP5142_1-EX-0000-2_3_4_54-16AIO_48AO_16DIO_16selDIO_CD-FF-01.bin  numconfig=-1  mode=Slave  externalClock=off  decimRtsi=0  calibIO=off  SampleTime=0  loadinport=-1
  OpCtrl : rtio_opalrt_common/OpCtrl  CtrlName='OpCtrl'  boardid=0  BitstreamFilename=VC707_2-EX-0001-2_3_2_20-48AIO16DIO16DIOSel-02-01.bin  numconfig=-1  mode=Master  externalClock=off  decimRtsi=0  calibIO=off  SampleTime=0  loadinport=-1  BoardType=VC707  SecondaryPresent=off  sync_type=Audio
  SEL751_01_DigitalAnalog_IO_OpBlocks : Subsystem
  Woodward Inputs : Subsystem
  Woodward Outputs - Diesel - Gen2 : Subsystem
  Woodward Outputs - NGCHP - Gen1 : Subsystem
  WoodwardBias : Outport
  wires:
  Bus Creator/1 -> [WoodwardBias]
  Memory1/1 -> WoodwardBias/1
  Bus Selector1/1 -> Woodward Outputs - NGCHP - Gen1/1(Gen1 MCB Status)  "<MCB_CB_Status>"
  [NGCHP_ScaledSignals] -> Bus Selector1/1
  [WoodwardBias] -> Woodward Outputs - NGCHP - Gen1/2(WoodwardBias)
  Woodward Outputs - NGCHP - Gen1/5(Gen1 MCB) -> Bus Creator2/5  "MCB_Ctrl"
  Woodward Outputs - Diesel - Gen2/1(Digital Inputs) -> Bus Creator1/1  "DIN"
  Woodward Outputs - NGCHP - Gen1/4(Gen1 GCB) -> Bus Creator2/4  "GCB_Crtl"
  Woodward Outputs - NGCHP - Gen1/3(Gen1 Fuel Enable) -> Bus Creator2/3  "FuelEnable"
  Woodward Outputs - NGCHP - Gen1/2(Gen1 Gov and AVR) -> Bus Creator2/2  "Gov_and_AVR"
  Woodward Outputs - NGCHP - Gen1/1(Digital Inputs) -> Bus Creator2/1  "DIN"
  Bus Creator2/1 -> Bus Creator3/1  "NGCHP_Gen1"
  Bus Creator3/1 -> Memory1/1
  Bus Creator1/1 -> Bus Creator3/2  "Diesel_Gen2"
  Woodward Outputs - Diesel - Gen2/5(Gen2 MCB) -> Bus Creator1/5  "MCB_Ctrl"
  Woodward Outputs - Diesel - Gen2/4(Gen2 GCB) -> Bus Creator1/4  "GCB_Crtl"
  Woodward Outputs - Diesel - Gen2/3(Gen2 Fuel Enable) -> Bus Creator1/3  "FuelEnable"
  Woodward Outputs - Diesel - Gen2/2(Gen2 Gov and AVR) -> Bus Creator1/2  "Gov_and_AVR"
  [Diesel_ScaledSignals] -> Bus Selector5/1
  [WoodwardBias] -> Woodward Outputs - Diesel - Gen2/2(WoodwardBias)
  Bus Selector5/1 -> Woodward Outputs - Diesel - Gen2/1(Gen2 MCB Status)  "<MCB_CB_Status>"
  Demux1/4 -> Bus Creator/4  "gen2_AVR_bias"
  Demux1/3 -> Bus Creator/3  "gen2_GOV_bias"
  Demux1/2 -> Bus Creator/2  "gen1_AVR_bias"
  Demux1/1 -> Bus Creator/1  "gen1_GOV_bias"
  GR1 B AIN (CH00-15)/1(Out1) -> Demux1/1
  Bus Selector4/5 -> Woodward Inputs/10(MPU2_speed)  "<scaled_speed>"
  Bus Selector4/4 -> Woodward Inputs/9(Mains2_Current)  "<scaled_mcb_current>"
  Bus Selector4/3 -> Woodward Inputs/8(Mains2_Voltage)  "<scaled_mcb_voltage>"
  Bus Selector4/2 -> Woodward Inputs/7(Generator2_Current)  "<scaled_gcb_current>"
  Bus Selector4/1 -> Woodward Inputs/6(Generator2_Voltage)  "<scaled_gcb_voltage>"
  [Diesel_ScaledSignals] -> Bus Selector4/1
  Bus Selector2/1 -> Woodward Inputs/1(Generator1_Voltage)  "<scaled_gcb_voltage>"
  Bus Selector2/2 -> Woodward Inputs/2(Generator1_Current)  "<scaled_gcb_current>"
  Bus Selector2/3 -> Woodward Inputs/3(Mains1_Voltage)  "<scaled_mcb_voltage>"
  Bus Selector2/4 -> Woodward Inputs/4(Mains1_Current)  "<scaled_mcb_current>"
  Bus Selector2/5 -> Woodward Inputs/5(MPU1_speed)  "<scaled_speed>"
  [NGCHP_ScaledSignals] -> Bus Selector2/1
  Bus Selector3/2 -> [Diesel_ScaledSignals]  "<Diesel_ScaledSignals>"
  Bus Selector3/1 -> [NGCHP_ScaledSignals]  "<NGCHP_ScaledSignals>"
  ScaledSignals/1 -> Bus Selector3/1
  SEL751_01_DigitalAnalog_IO_OpBlocks/1(SEL751-01_LogicTrip) -> Bus Creator3/3  "SEL751-F1_LogicTrip"
  [SEL751_F1_ScaledSignals] -> SEL751_01_DigitalAnalog_IO_OpBlocks/1(SEL751-01_ScaledSignals)
  Bus Selector3/3 -> [SEL751_F1_ScaledSignals]  "<SEL751_F1_ScaledSignals>"

== system MINI_BANSHEE_bckup/SS_F3/HWController_3.5MVA_NGCHP ==
  note: Copyright (c) 2016 Massachusetts Institute of Technology
      | Permission is hereby granted, free of charge, to any person obtaining a copy of this software and associated documentation files (the "Software"), to deal
      | in the Software without restriction, including without limitation the rights to use, copy, modify, merge, publish, distribute, sublicense, and/or sell copies of the
      | Software, and to permit persons to whom the Software is furnished to do so, subject to the following conditions:
      |
      | THE SOFTWARE IS PROVIDED "AS IS", WITHOUT WARRANTY OF ANY KIND, EXPRESS OR IMPLIED, INCLUDING BUT NOT LIMITED TO THE
      | WARRANTIES OF MERCHANTABILITY, FITNESS FOR A PARTICULAR PURPOSE AND NONINFRINGEMENT. IN NO EVENT SHALL THE AUTHORS
      | OR COPYRIGHT HOLDERS BE LIABLE FOR ANY CLAIM, DAMAGES OR OTHER LIABILITY, WHETHER IN AN ACTION OF CONTRACT, TORT OR
      | OTHERWISE, ARISING FROM, OUT OF OR IN CONNECTION WITH THE SOFTWARE OR THE USE OR OTHER DEALINGS IN THE SOFTWARE
  In1 : Inport
  In2 : Inport  Port=2
  HWControllerBias : Inport  Port=3
  Bus Creator2 : BusCreator  Inputs=6
  Bus Selector6 : BusSelector  OutputSignals=Heat Recovered; MBtu/hr
  Bus Selector7 : BusSelector  OutputSignals=TempActual,HeatFromBoiler MBtu/hr,CHPHeatContribution MBtu/hr,Thermal data.Heat Recovered; MBtu/hr,Thermal data.CO2 lbm/hr,Boiler_Nm^3/hr ,Boiler lbm/hr CO2
  CHPThermalModel : CHP_Model_lib/CHPThermalModel  SIM_HIL=SIM_HIL
  Demux : Demux  Outputs=2
  HWController_NG_Generator : HWController_NGCHP_Genset_3p5MVA_lib/HWController_NG_Generator
  Modbus device : rtio_generic_modbus/Modbus device  conf_name=CHP_slave_cfg.opal  conf_name_mask=CHP_slave_cfg.xls  sample_time=Ts
  Mux1 : Mux  Inputs=7
  A : PMIOPort  Tag=A  Port=1  Side=Right
      settings: AttributesFormatString=A
  B : PMIOPort  Port=2  Side=Right
  C : PMIOPort  Port=3  Side=Right
  Out1 : Outport
  Generator Data : Outport  Port=2
  GCB Control : Outport  Port=3
  wires:
  Bus Selector7/6 -> Mux1/6  "<Boiler_Nm^3/hr >"
  Bus Selector7/7 -> Mux1/7  "<Boiler lbm/hr CO2 >"
  CHPThermalModel/5 -> Bus Creator2/6
  CHPThermalModel/4 -> Bus Creator2/5
  HWControllerBias/1 -> HWController_NG_Generator/1
  HWController_NG_Generator/3 -> [HeatRec_MBtuhr]  "Thermal data"
  Bus Selector7/3 -> Mux1/3  "<CHPHeatContribution MBtu/hr>"
  CHPThermalModel/1 -> Bus Creator2/2  "TempActual"
  Demux/2 -> CHPThermalModel/4
  CHPThermalModel/2 -> Bus Creator2/3
  Bus Selector7/2 -> Mux1/2  "<HeatFromBoiler MBtu/hr>"
  Bus Selector7/5 -> Mux1/5  "<CO2 lbm/hr>"
  Bus Selector7/4 -> Mux1/4  "<Heat Recovered; MBtu/hr>"
  Bus Selector7/1 -> Mux1/1  "<TempActual>"
  In1/1 -> CHPThermalModel/2
  Mux1/1 -> Modbus device/4
  Demux/1 -> CHPThermalModel/3
  CHPThermalModel/3 -> Bus Creator2/4
  [HeatRec_MBtuhr] -> Bus Selector6/1, Bus Creator2/1  "Thermal data"
  Modbus device/2 -> Demux/1
  HWController_NG_Generator/1 -> Generator Data/1
  HWController_NG_Generator/2 -> GCB Control/1
  Bus Selector6/1 -> CHPThermalModel/1  "<Heat Recovered; MBtu/hr>"
  Bus Creator2/1 -> Out1/1, Bus Selector7/1  "CHPData"
  In2/1 -> CHPThermalModel/5  "CHP_SIM_Cmds"
  connections:
  HWController_NG_Generator/RConn3 -- C/RConn1
  HWController_NG_Generator/RConn2 -- B/RConn1
  HWController_NG_Generator/RConn1 -- A/RConn1

== system MINI_BANSHEE_bckup/SS_F3_RELAY_HOUSING/Load_Profiles ==
  note: % Copyright (c) 2016 Massachusetts Institute of Technology
      | % Permission is hereby granted, free of charge, to any person obtaining a copy of this
      | % software and associated documentation files (the "Software"), to deal in the Software
      | % without restriction, including without limitation the rights to use, copy, modify,
      | % merge, publish, distribute, sublicense, and/or sell copies of the Software, and to
      | % permit persons to whom the Software is furnished to do so, subject to the following
      | % conditions:
      | %
      | %
      | % The above copyright notice and this permission notice shall be included in
      | % all copies or substantial portions of the Software.
      | %
      | % THE SOFTWARE IS PROVIDED "AS IS", WITHOUT WARRANTY OF ANY KIND, EXPRESS OR IMPLIED,
      | % INCLUDING BUT NOT LIMITED TO THE WARRANTIES OF MERCHANTABILITY, FITNESS FOR A
      | % PARTICULAR PURPOSE AND NONINFRINGEMENT. IN NO EVENT SHALL THE AUTHORS OR COPYRIGHT
      | % HOLDERS BE LIABLE FOR ANY CLAIM, DAMAGES OR OTHER LIABILITY, WHETHER IN AN ACTION
      | % OF CONTRACT, TORT OR OTHERWISE, ARISING FROM, OUT OF OR IN CONNECTION WITH THE
      | % SOFTWARE OR THE USE OR OTHER DEALINGS IN THE SOFTWARE.
      | %
      | %
      | %%
  note: Stop_index = length of data - 1 to data chopping
  Bus Creator2 : BusCreator  Inputs=2
  Demux1 : Demux  Outputs=6
  Demux2 : Demux  Outputs=6
  "Interpolation " : Constant
  Mux : Mux  Inputs=6
  OpFromFile : rtlab/DataLogging/OpFromFile  filename_mode=Static (same filename all the time)  reload_mode=Next time model is paused (Real-Time)  init_file_id=0  filename=NONSHEDDABLE.mat  rtpath='./'  nrtpath='.\'  sample_time=0
  OpFromFile1 : rtlab/DataLogging/OpFromFile  filename_mode=Static (same filename all the time)  reload_mode=Next time model is paused (Real-Time)  init_file_id=0  filename=SHEDDABLE.mat  rtpath='./'  nrtpath='.\'  sample_time=0
  "Repetative " : Constant
  "Start_Index " : Constant
  "State " : Constant
  "Stop_Index " : Constant  Value=2000-1
  "Time_Scale_Factor " : Constant
  LOAD_OUT : Outport
  wires:
  Mux/1 -> Demux2/1, Demux1/1
  Bus Creator2/1 -> LOAD_OUT/1
  Demux1/1 -> OpFromFile/1
  Demux1/2 -> OpFromFile/2
  Demux1/3 -> OpFromFile/3
  Demux2/6 -> OpFromFile1/6
  Demux2/4 -> OpFromFile1/4
  Demux2/3 -> OpFromFile1/3
  Demux1/4 -> OpFromFile/4
  Demux2/5 -> OpFromFile1/5
  Demux2/2 -> OpFromFile1/2
  Demux2/1 -> OpFromFile1/1
  Demux1/5 -> OpFromFile/5
  Demux1/6 -> OpFromFile/6
  "Repetative "/1 -> Mux/2
  "State "/1 -> Mux/1
  OpFromFile/2 -> Bus Creator2/1  "NONSHEDDABLE"
  "Start_Index "/1 -> Mux/3
  OpFromFile1/2 -> Bus Creator2/2  "SHEDDABLE"
  "Time_Scale_Factor "/1 -> Mux/5
  "Stop_Index "/1 -> Mux/4
  "Interpolation "/1 -> Mux/6

== system MINI_BANSHEE_bckup/SC_ctrl/Overall/currents ==
  F1 : Inport
  F2 : Inport  Port=2
  F3 : Inport  Port=3
  1ph_rms1 : Subsystem
  1ph_rms10 : Subsystem
  1ph_rms11 : Subsystem
  1ph_rms12 : Subsystem
  1ph_rms13 : Subsystem
  1ph_rms14 : Subsystem
  1ph_rms15 : Subsystem
  1ph_rms2 : Subsystem
  1ph_rms3 : Subsystem
  1ph_rms4 : Subsystem
  1ph_rms5 : Subsystem
  1ph_rms6 : Subsystem
  1ph_rms7 : Subsystem
  1ph_rms8 : Subsystem
  1ph_rms9 : Subsystem
  Bus Selector : BusSelector  OutputSignals=F1_CB_1.m.Iabc,F1_CB_2.m.Iabc,F1_CB_3.m.Iabc,F1_CB_6.m.Iabc,F1_CB_10.m.Iabc
  Bus Selector1 : BusSelector  OutputSignals=F2_CB_1.m.Iabc,F2_CB_2.m.Iabc,F2_CB_3.m.Iabc,F2_CB_7.m.Iabc,F2_CB_14.m.Iabc,F2_CB_15.m.Iabc
  Bus Selector2 : BusSelector  OutputSignals=F3_CB_1.m.Iabc,F3_CB_2.m.Iabc,F3_CB_3.m.Iabc,F3_CB_4.m.Iabc
  Mux : Mux  Inputs=5
  Mux1 : Mux  Inputs=6
  Mux2 : Mux
  RMS_Calculator : Subsystem
  RMS_Calculator1 : Subsystem
  RMS_Calculator2 : Subsystem
  oF1 : Outport
  oF2 : Outport  Port=2
  oF3 : Outport  Port=3
  wires:
  Mux/1 -> RMS_Calculator/1(Signal)  "F1"
  Mux1/1 -> RMS_Calculator1/1(Signal)  "F2"
  Mux2/1 -> RMS_Calculator2/1(Signal)  "F3"
  Bus Selector/5 -> 1ph_rms3/1(i)  "<Iabc>"
  Bus Selector/4 -> 1ph_rms4/1(i)  "<Iabc>"
  Bus Selector/3 -> 1ph_rms2/1(i)  "<Iabc>"
  Bus Selector/2 -> 1ph_rms1/1(i)  "<Iabc>"
  Bus Selector/1 -> 1ph_rms6/1(i)  "<Iabc>"
  Bus Selector1/4 -> 1ph_rms9/1(i)  "<Iabc>"
  Bus Selector1/5 -> 1ph_rms13/1(i)  "<Iabc>"
  Bus Selector1/3 -> 1ph_rms8/1(i)  "<Iabc>"
  Bus Selector1/6 -> 1ph_rms10/1(i)  "<Iabc>"
  Bus Selector1/2 -> 1ph_rms7/1(i)  "<Iabc>"
  Bus Selector1/1 -> 1ph_rms5/1(i)  "<Iabc>"
  Bus Selector2/4 -> 1ph_rms15/1(i)  "<Iabc>"
  Bus Selector2/2 -> 1ph_rms12/1(i)  "<Iabc>"
  Bus Selector2/3 -> 1ph_rms11/1(i)  "<Iabc>"
  Bus Selector2/1 -> 1ph_rms14/1(i)  "<Iabc>"
  1ph_rms6/1(o) -> Mux/1
  1ph_rms1/1(o) -> Mux/2
  1ph_rms2/1(o) -> Mux/3
  1ph_rms3/1(o) -> Mux/5
  1ph_rms4/1(o) -> Mux/4
  1ph_rms5/1(o) -> Mux1/1
  1ph_rms7/1(o) -> Mux1/2
  1ph_rms8/1(o) -> Mux1/3
  1ph_rms9/1(o) -> Mux1/4
  1ph_rms14/1(o) -> Mux2/1
  1ph_rms13/1(o) -> Mux1/5
  1ph_rms10/1(o) -> Mux1/6
  1ph_rms12/1(o) -> Mux2/2
  1ph_rms11/1(o) -> Mux2/3
  1ph_rms15/1(o) -> Mux2/4
  RMS_Calculator/1(RMS_Signal) -> oF1/1
  RMS_Calculator1/1(RMS_Signal) -> oF2/1
  RMS_Calculator2/1(RMS_Signal) -> oF3/1
  F1/1 -> Bus Selector/1
  F2/1 -> Bus Selector1/1
  F3/1 -> Bus Selector2/1

== system MINI_BANSHEE_bckup/SC_ctrl/Overall/voltages ==
  F1 : Inport
  F2 : Inport  Port=2
  F3 : Inport  Port=3
  Bus Selector : BusSelector  OutputSignals=F1_CB_1.m.Vpu,F1_CB_2.m.Vpu,F1_CB_3.m.Vpu,F1_CB_4.m.Vpu,F1_CB_5.m.Vpu,F1_CB_6.m.Vpu,F1_CB_7.m.Vpu,F1_CB_8.m.Vpu,F1_CB_9.m.Vpu,F1_CB_10.m.Vpu,F1_CB_11.m.Vpu,F1_CB_12.m.Vpu,F1_CB_13.m.Vpu,F1_CB_14.m.Vpu
  Bus Selector1 : BusSelector  OutputSignals=F2_CB_1.m.Vpu,F2_CB_2.m.Vpu,F2_CB_3.m.Vpu,F2_CB_4.m.Vpu,F2_CB_5.m.Vpu,F2_CB_6.m.Vpu,F2_CB_7.m.Vpu,F2_CB_8.m.Vpu,F2_CB_9.m.Vpu,F2_CB_10.m.Vpu,F2_CB_11.m.Vpu,F2_CB_12.m.Vpu,F2_CB_13.m.Vpu,F2_CB_14.m.Vpu,F2_CB_15.m.Vpu,F2_CB_16.m.Vpu,F2_CB_17.m.Vpu,F2_CB_18.m.Vpu,F2_CB_19.m.Vpu
  Bus Selector2 : BusSelector  OutputSignals=F3_CB_1.m.Vpu,F3_CB_2.m.Vpu,F3_CB_3.m.Vpu,F3_CB_4.m.Vpu,F3_CB_5.m.Vpu,F3_CB_6.m.Vpu,F3_CB_7.m.Vpu,F3_CB_8.m.Vpu,F3_CB_9.m.Vpu
  Mux : Mux  Inputs=14
  Mux1 : Mux  Inputs=19
  Mux2 : Mux  Inputs=9
  oF1 : Outport
  oF2 : Outport  Port=2
  oF3 : Outport  Port=3
  wires:
  Mux/1 -> oF1/1  "F1"
  F1/1 -> Bus Selector/1
  Mux1/1 -> oF2/1  "F2"
  F2/1 -> Bus Selector1/1
  Mux2/1 -> oF3/1  "F3"
  F3/1 -> Bus Selector2/1
  Bus Selector/14 -> Mux/14  "<Vpu>"
  Bus Selector/6 -> Mux/6  "<Vpu>"
  Bus Selector/5 -> Mux/5  "<Vpu>"
  Bus Selector/10 -> Mux/10  "<Vpu>"
  Bus Selector/4 -> Mux/4  "<Vpu>"
  Bus Selector/9 -> Mux/9  "<Vpu>"
  Bus Selector/7 -> Mux/7  "<Vpu>"
  Bus Selector/2 -> Mux/2  "<Vpu>"
  Bus Selector/1 -> Mux/1  "<Vpu>"
  Bus Selector/3 -> Mux/3  "<Vpu>"
  Bus Selector/13 -> Mux/13  "<Vpu>"
  Bus Selector/12 -> Mux/12  "<Vpu>"
  Bus Selector/11 -> Mux/11  "<Vpu>"
  Bus Selector/8 -> Mux/8  "<Vpu>"
  Bus Selector1/19 -> Mux1/19  "<Vpu>"
  Bus Selector1/18 -> Mux1/18  "<Vpu>"
  Bus Selector1/7 -> Mux1/7  "<Vpu>"
  Bus Selector1/10 -> Mux1/10  "<Vpu>"
  Bus Selector1/11 -> Mux1/11  "<Vpu>"
  Bus Selector1/2 -> Mux1/2  "<Vpu>"
  Bus Selector1/13 -> Mux1/13  "<Vpu>"
  Bus Selector1/14 -> Mux1/14  "<Vpu>"
  Bus Selector1/15 -> Mux1/15  "<Vpu>"
  Bus Selector1/6 -> Mux1/6  "<Vpu>"
  Bus Selector1/4 -> Mux1/4  "<Vpu>"
  Bus Selector1/3 -> Mux1/3  "<Vpu>"
  Bus Selector1/1 -> Mux1/1  "<Vpu>"
  Bus Selector1/5 -> Mux1/5  "<Vpu>"
  Bus Selector1/8 -> Mux1/8  "<Vpu>"
  Bus Selector1/12 -> Mux1/12  "<Vpu>"
  Bus Selector1/16 -> Mux1/16  "<Vpu>"
  Bus Selector1/17 -> Mux1/17  "<Vpu>"
  Bus Selector1/9 -> Mux1/9  "<Vpu>"
  Bus Selector2/5 -> Mux2/5  "<Vpu>"
  Bus Selector2/4 -> Mux2/4  "<Vpu>"
  Bus Selector2/6 -> Mux2/6  "<Vpu>"
  Bus Selector2/3 -> Mux2/3  "<Vpu>"
  Bus Selector2/7 -> Mux2/7  "<Vpu>"
  Bus Selector2/8 -> Mux2/8  "<Vpu>"
  Bus Selector2/2 -> Mux2/2  "<Vpu>"
  Bus Selector2/9 -> Mux2/9  "<Vpu>"
  Bus Selector2/1 -> Mux2/1  "<Vpu>"

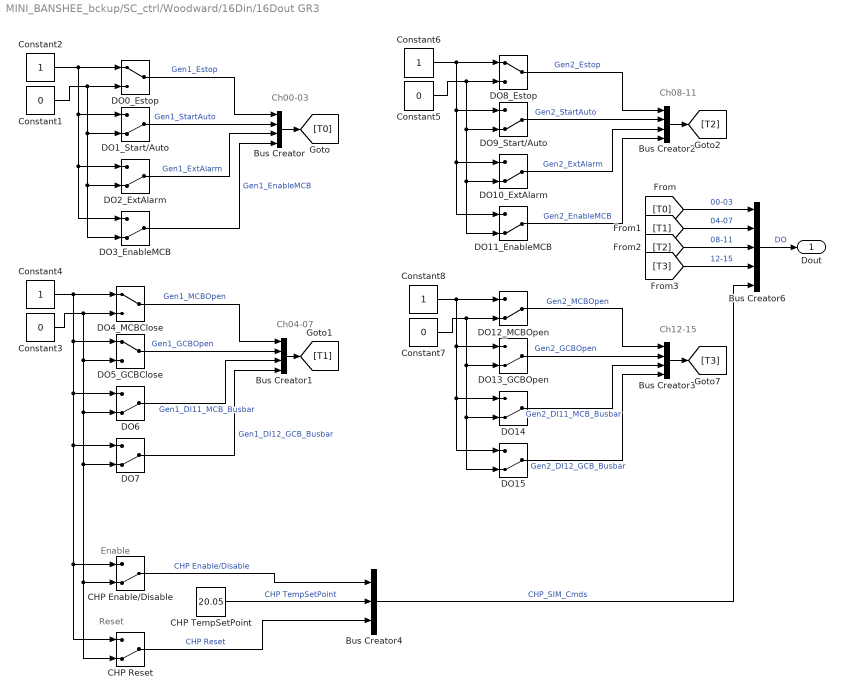
== system MINI_BANSHEE_bckup/SC_ctrl/Woodward/16Din/16Dout GR3 ==
  note: Ch00-03
  note: Ch04-07
  note: Ch08-11
  note: Ch12-15
  note: Enable
  note: Reset
  Bus Creator{,1..3} (4 alike) : BusCreator
  Bus Creator4 : BusCreator  Inputs=3
  Bus Creator6 : BusCreator  Inputs=5
  CHP Enable/Disable : ManualSwitch  CurrentSetting=0
  CHP Reset : ManualSwitch  CurrentSetting=0
  CHP TempSetPoint : Constant  Value=20.05
  Constant{1,3,5,7} (4 alike) : Constant  Value=0
  Constant{2,4,6,8} (4 alike) : Constant
  DO0_Estop : ManualSwitch
  DO10_ExtAlarm : ManualSwitch  CurrentSetting=0
  DO11_EnableMCB : ManualSwitch  CurrentSetting=0
  DO12_MCBOpen : ManualSwitch  CurrentSetting=0
  DO13_GCBOpen : ManualSwitch  CurrentSetting=0
  DO{6..7,14..15} (4 alike) : ManualSwitch  CurrentSetting=0
  DO1_Start/Auto : ManualSwitch  CurrentSetting=0
  DO2_ExtAlarm : ManualSwitch  CurrentSetting=0
  DO3_EnableMCB : ManualSwitch  CurrentSetting=0
  DO4_MCBClose : ManualSwitch
  DO5_GCBClose : ManualSwitch
  DO8_Estop : ManualSwitch
  DO9_Start/Auto : ManualSwitch  CurrentSetting=0
  Dout : Outport
  wires:
  Bus Creator4/1 -> Bus Creator6/5  "CHP_SIM_Cmds"
  CHP Reset/1 -> Bus Creator4/3  "CHP Reset"
  CHP TempSetPoint/1 -> Bus Creator4/2  "CHP TempSetPoint"
  CHP Enable/Disable/1 -> Bus Creator4/1  "CHP Enable/Disable"
  Bus Creator6/1 -> Dout/1  "DO"
  Constant2/1 -> DO0_Estop/1, DO1_Start/Auto/1, DO3_EnableMCB/1, DO2_ExtAlarm/1
  Constant1/1 -> DO0_Estop/2, DO1_Start/Auto/2, DO3_EnableMCB/2, DO2_ExtAlarm/2
  DO0_Estop/1 -> Bus Creator/1  "Gen1_Estop"
  DO1_Start/Auto/1 -> Bus Creator/2  "Gen1_StartAuto"
  DO2_ExtAlarm/1 -> Bus Creator/3  "Gen1_ExtAlarm"
  DO3_EnableMCB/1 -> Bus Creator/4  "Gen1_EnableMCB"
  Constant4/1 -> DO6/1, DO7/1, CHP Enable/Disable/1, CHP Reset/1, DO5_GCBClose/1, DO4_MCBClose/1
  Constant3/1 -> DO6/2, CHP Enable/Disable/2, CHP Reset/2, DO7/2, DO5_GCBClose/2, DO4_MCBClose/2
  DO4_MCBClose/1 -> Bus Creator1/1  "Gen1_MCBOpen"
  DO5_GCBClose/1 -> Bus Creator1/2  "Gen1_GCBOpen"
  DO6/1 -> Bus Creator1/3  "Gen1_DI11_MCB_Busbar"
  DO7/1 -> Bus Creator1/4  "Gen1_DI12_GCB_Busbar"
  Constant6/1 -> DO8_Estop/1, DO9_Start/Auto/1, DO11_EnableMCB/1, DO10_ExtAlarm/1
  Constant5/1 -> DO8_Estop/2, DO9_Start/Auto/2, DO11_EnableMCB/2, DO10_ExtAlarm/2
  DO8_Estop/1 -> Bus Creator2/1  "Gen2_Estop"
  DO9_Start/Auto/1 -> Bus Creator2/2  "Gen2_StartAuto"
  DO10_ExtAlarm/1 -> Bus Creator2/3  "Gen2_ExtAlarm"
  DO11_EnableMCB/1 -> Bus Creator2/4  "Gen2_EnableMCB"
  Constant8/1 -> DO14/1, DO15/1, DO13_GCBOpen/1, DO12_MCBOpen/1
  Constant7/1 -> DO14/2, DO15/2, DO13_GCBOpen/2, DO12_MCBOpen/2
  DO12_MCBOpen/1 -> Bus Creator3/1  "Gen2_MCBOpen"
  DO13_GCBOpen/1 -> Bus Creator3/2  "Gen2_GCBOpen"
  DO14/1 -> Bus Creator3/3  "Gen2_DI11_MCB_Busbar"
  DO15/1 -> Bus Creator3/4  "Gen2_DI12_GCB_Busbar"
  Bus Creator/1 -> [T0]
  Bus Creator1/1 -> [T1]
  Bus Creator3/1 -> [T3]
  Bus Creator2/1 -> [T2]
  [T0] -> Bus Creator6/1  "00-03"
  [T1] -> Bus Creator6/2  "04-07"
  [T2] -> Bus Creator6/3  "08-11"
  [T3] -> Bus Creator6/4  "12-15"

== system MINI_BANSHEE_bckup/SM_UtilityService/HWCtrl_IOs/GR1 B AIN (CH00-15) ==
  AnalogIn : rtio_opalrt_common/AnalogIn  CtrlName='OpCtrl'  portNb=1  FcnNos=Slot 1 Module B Subsection 1  size=16  maxcount=8  count=8  numchan=8  sampleTime=0
      settings: AttributesFormatString=%<CtrlName>
  AnalogIn1 : rtio_opalrt_common/AnalogIn  CtrlName='OpCtrl'  portNb=2  FcnNos=Slot 1 Module B Subsection 2  size=16  maxcount=8  count=8  numchan=8  sampleTime=0
      settings: AttributesFormatString=%<CtrlName>
  Mux6 : Mux  Inputs=2
  Terminator2 : Terminator
  Terminator3 : Terminator
  Out1 : Outport
  wires:
  Mux6/1 -> Out1/1
  AnalogIn1/2 -> Terminator3/1
  AnalogIn/2 -> Terminator2/1
  AnalogIn1/1 -> Mux6/2
  AnalogIn/1 -> Mux6/1

== system MINI_BANSHEE_bckup/SM_UtilityService/HWCtrl_IOs/SEL751_01_DigitalAnalog_IO_OpBlocks ==
  note: Copyright (c) 2016 Massachusetts Institute of Technology
      | Permission is hereby granted, free of charge, to any person obtaining a copy of this software and associated documentation files (the "Software"), to deal
      | in the Software without restriction, including without limitation the rights to use, copy, modify, merge, publish, distribute, sublicense, and/or sell copies of the
      | Software, and to permit persons to whom the Software is furnished to do so, subject to the following conditions:
      |
      | THE SOFTWARE IS PROVIDED "AS IS", WITHOUT WARRANTY OF ANY KIND, EXPRESS OR IMPLIED, INCLUDING BUT NOT LIMITED TO THE
      | WARRANTIES OF MERCHANTABILITY, FITNESS FOR A PARTICULAR PURPOSE AND NONINFRINGEMENT. IN NO EVENT SHALL THE AUTHORS
      | OR COPYRIGHT HOLDERS BE LIABLE FOR ANY CLAIM, DAMAGES OR OTHER LIABILITY, WHETHER IN AN ACTION OF CONTRACT, TORT OR
      | OTHERWISE, ARISING FROM, OUT OF OR IN CONNECTION WITH THE SOFTWARE OR THE USE OR OTHER DEALINGS IN THE SOFTWARE
  note: When the system uses the simulated
      | Secondary Controller the digital I/O
      | should be disabled.
  SEL751-01_ScaledSignals : Inport
  Bus Creator4 : BusCreator  Inputs=2
  Bus Selector4 : BusSelector  OutputSignals=To DigitalOut_to_SEL-751,To AnalogOut_to_SEL-751
  Data Type Conversion{,1..3} (4 alike) : DataTypeConversion
  Demux6 : Demux  Outputs=8
  OP5142EX1 AnalogOut1 : rtio_opalrt_op5142ex1/OP5142EX1 AnalogOut  CtrlName='OP5142EX1 Ctrl'  portNb=1  FcnNos=Slot 1 Module A Subsection 1  size=16  maxcount=8  count=8  numchan=8  israngeinput=off  voltagerange=[-16 ... 16]  slot=0  side=0  mismatch=0  slotside=Slot_1_Module_A
      settings: AttributesFormatString=%<CtrlName>
  OP5142EX1 DigitalIn : rtio_opalrt_op5142ex1/OP5142EX1 DigitalIn  CtrlName='OP5142EX1 Ctrl'  portNb=3  FcnNos=Slot 4 Module A Subsection 1  size=1  maxcount=8  count=8  sampleTime=Ts  numchan=8
      settings: AttributesFormatString=%<CtrlName>
  OP5142EX1 DigitalOut1 : rtio_opalrt_op5142ex1/OP5142EX1 DigitalOut  CtrlName='OP5142EX1 Ctrl'  portNb=9  FcnNos=Slot 4 Module B Subsection 1  size=1  maxcount=8  count=8  numchan=8
      settings: AttributesFormatString=%<CtrlName>
  S-R Flip-Flop : simulink_extras/Flip Flops/S-R Flip-Flop  initial_condition=1
  Terminator : Terminator
  Terminator1 : Terminator
  Terminator2 : Terminator
  SEL751-01_LogicTrip : Outport
  wires:
  S-R Flip-Flop/2 -> Data Type Conversion3/1  "Logic_reset"
  S-R Flip-Flop/1 -> Data Type Conversion2/1  "Logic_trip"
  Bus Creator4/1 -> SEL751-01_LogicTrip/1
  Data Type Conversion2/1 -> Bus Creator4/1  "Logic_trip"
  Data Type Conversion1/1 -> S-R Flip-Flop/2
  OP5142EX1 DigitalIn/1 -> Demux6/1
  SEL751-01_ScaledSignals/1 -> Bus Selector4/1
  OP5142EX1 DigitalIn/2 -> Terminator2/1
  Bus Selector4/1 -> OP5142EX1 DigitalOut1/1  "<To DigitalOut_to_SEL-751>"
  Bus Selector4/2 -> OP5142EX1 AnalogOut1/1  "<To AnalogOut_to_SEL-751>"
  Data Type Conversion/1 -> S-R Flip-Flop/1
  Data Type Conversion3/1 -> Bus Creator4/2  "Logic_reset"
  Demux6/1 -> Data Type Conversion/1  "OUT103 Brkr trip"
  Demux6/2 -> Data Type Conversion1/1  "OUT102 Brkr reset"
  OP5142EX1 AnalogOut1/1 -> Terminator/1
  OP5142EX1 DigitalOut1/1 -> Terminator1/1
